simulink model "resistB_Lineal"  (R2018a)
settings: Solver=VariableStepAuto  StartTime=0.0  StopTime=100  MaxStep=0.05  RelTol=1e-3
values from neighbouring files (symbols this model uses):
  A = [S.A zeros(n,p); -S.C eye(p)]    [poles_int.m]
  B = [S.B; zeros(p,m)]    [poles_int.m]
  ro = 0.0683    [LaplaceAzeta.m]    (also in discretizacion.m = 0.0683238685925)
  so = 0.3356    [LaplaceAzeta.m]    (also in discretizacion.m = 0.335599308431)
undefined symbols (not defined in the file or in its folder): C, D, kp, Kp, Td, Ti
libraries: simulink x2
settings Model: Creator=posoriol1  LastModifiedBy=posoriol1
settings CodeAppCC: StateflowObjectComments=on

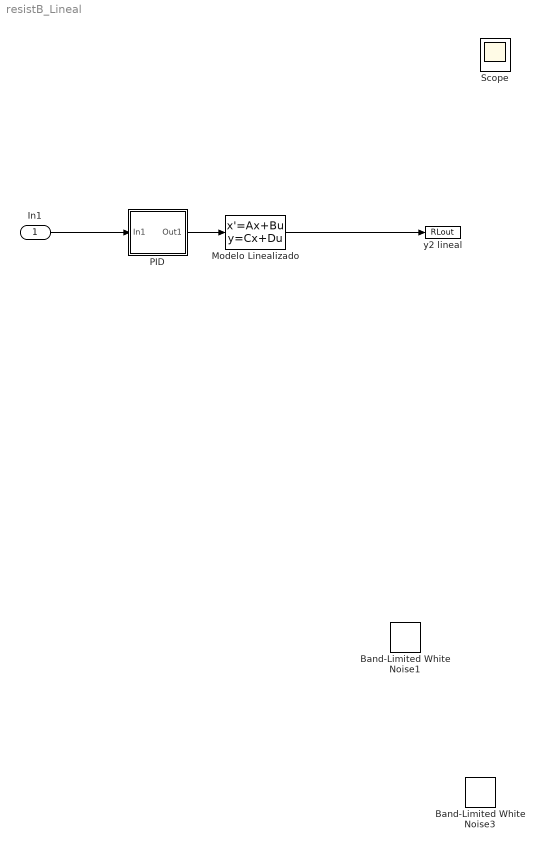
== system resistB_Lineal ==
  In1 : Inport
  Band-Limited White Noise1 : simulink/Sources/Band-Limited White Noise  Cov=[0.0000005]  Ts=0.3  seed=[11558]
  Band-Limited White Noise3 : simulink/Sources/Band-Limited White Noise  Cov=[0.0000005]  Ts=0.3  seed=[11558]
  "Modelo Linealizado " : StateSpace  A=A  B=B  C=C  D=D  InitialCondition=[so ro]
  PID : Subsystem  mask{par=[kp,Ti,Td,5]}
      mask prompts: par "[kp Ti Td N]"
      mask init:
      | kp = par(1);
      | Ti = par(2);
      | Td = par(3);
      | N = par(4);
  Scope : Scope  NumInputPorts=2
  y2 lineal : ToWorkspace  VariableName=RLout  SampleTime=-1
  wires:
  "Modelo Linealizado "/1 -> y2 lineal/1
  In1/1 -> PID/1(In1)
  PID/1(Out1) -> "Modelo Linealizado "/1

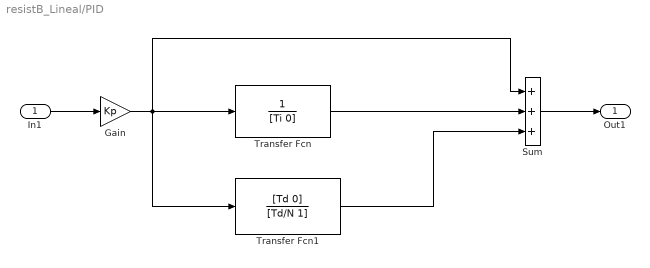
== system resistB_Lineal/PID ==
  In1 : Inport
  Gain : Gain  Gain=Kp
  Sum : Sum  Inputs=+++
  Transfer Fcn : TransferFcn  Denominator=[Ti 0]
  Transfer Fcn1 : TransferFcn  Numerator=[Td 0]  Denominator=[Td/N 1]
  Out1 : Outport
  wires:
  In1/1 -> Gain/1
  Gain/1 -> Sum/1, Transfer Fcn1/1, Transfer Fcn/1
  Transfer Fcn/1 -> Sum/2
  Transfer Fcn1/1 -> Sum/3
  Sum/1 -> Out1/1
